simulink model "VirtualVehicle_lab2"  (R2021a)
settings: Solver=VariableStepAuto  StartTime=0.0  StopTime=30  MaxStep=0.002  RelTol=1e-3
libraries: PlantLibrary x1
settings Model: Creator=Rocksmithed  LastModifiedBy=Rocksmithed
settings ExplorerConfigSet: InternalSimMechanicsExplorerSettings="<ExplorerConfiguration><canonicalview>default</canonicalview><AnimationSetting><BasePlaybackSpeed>1.0</BasePlaybackSpeed><PlaybackSpeedFactor>1.0</PlaybackSpeedFactor></AnimationSetting><TilePanel><TileInfo><Tiles Columns=\"1\" Count=\"2\" Rows=\"2\"><Column Weight=\"1\"/><Row Weight=\"0.4997\"/><Row Weight=\"0.5003\"/><Tile Height=\"1\" Width=\"1\" X=\"0\" Y=\"0\"/><Tile Height=\"1\" Width=\"1\" X=\"0\" Y=\"1\"/></Tiles></TileInfo><SceneInfo><SceneViewer><BGColor><R>0.800000011920928955</R><G>0.800000011920928955</G><B>0.800000011920928955</B></BGColor><Camera><DoPerspective>on</DoPerspective><Position><X>442.389269826050509</X><Y>-6</Y><Z>6.75</Z></Position><Center><X>441.815693389699447</X><Y>-5.37249312840286741</Y><Z>6.22345921548163616</Z></Center><Up><X>0</X><Y>0</Y><Z>1</Z></Up><ViewLimDist>1</ViewLimDist><YLim>0.466307658154998583</YLim><XLim>1.37909215060664225</XLim></Camera></SceneViewer><SceneViewer><BGColor><R>0.800000011920928955</R><G>0.800000011920928955</G><B>0.800000011920928955</B></BGColor><Camera><DoPerspective>on</DoPerspective><Position><X>435.489269826050531</X><Y>-15</Y><Z>8.3066149444976863e-16</Z></Position><Center><X>435.489269826050531</X><Y>-14</Y><Z>6.08616889524737322e-16</Z></Center><Up><X>0</X><Y>0</Y><Z>1</Z></Up><ViewLimDist>1</ViewLimDist><YLim>0.466307658154998583</YLim><XLim>1.37741849508406133</XLim></Camera></SceneViewer></SceneInfo></TilePanel><MechEditorPanel><Cameras><Camera><Id>Camera1</Id><Value><Name>Camera1</Name><NativeCamera><PositionTrackingFeature>Vehicle_and_road.camera.R</PositionTrackingFeature><CenterTrackingFeature>Vehicle_and_road.camera.R</CenterTrackingFeature><UpVectorTrackingFeature>Vehicle_and_road.World_Frame.W</UpVectorTrackingFeature><CenterTrackingOrigin>off</CenterTrackingOrigin><CenterTrackingDirection>-Z</CenterTrackingDirection><UpVectorTrackingDirection>+Z</UpVectorTrackingDirection></NativeCamera></Value></Camera><Camera><Id>Camera2</Id><Value><Name>Camera2</Name><NativeCamera><PositionTrackingFeature>Vehicle_and_road.camera1.R</PositionTrackingFeature><CenterTrackingFeature>Vehicle_and_road.camera1.R</CenterTrackingFeature><UpVectorTrackingFeature>Vehicle_and_road.World_Frame.W</UpVectorTrackingFeature><CenterTrackingOrigin>off</CenterTrackingOrigin><CenterTrackingDirection>-Z</CenterTrackingDirection><UpVectorTrackingDirection>+Z</UpVectorTrackingDirection></NativeCamera></Value></Camera></Cameras><GfxPanelCameraMap><MapElement CameraMLId=\"Camera1\" GfxPanelIndex=\"0\"/><MapElement CameraMLId=\"Camera2\" GfxPanelIndex=\"1\"/></GfxPanelCameraMap><VideoCreator><PlaybackSpeedRatio>1.0</PlaybackSpeedRatio><FrameRate>30</FrameRate><VideoFormat>Motion JPEG AVI</VideoFormat><FrameSize>auto</FrameSize></VideoCreator></MechEditorPanel></ExplorerConfiguration>"

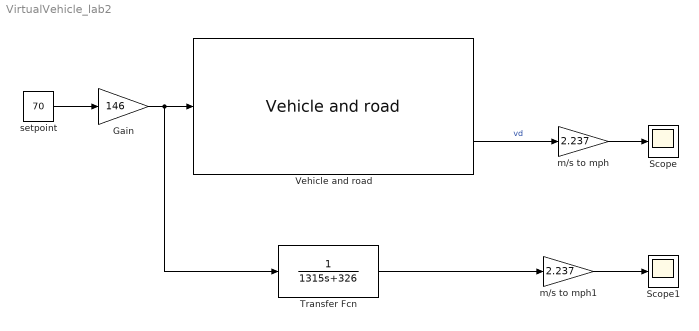
== system VirtualVehicle_lab2 ==
  Gain : Gain  Gain=146
  Scope : Scope
  Scope1 : Scope
  Transfer Fcn : TransferFcn  Denominator=[1315 326]
  Vehicle and road : PlantLibrary/Vehicle and road  MaxF=14800.0  brkok=on  dtype=none  randbumps=on  h=50  bumpspace=68.0
  m/s to mph : Gain  Gain=2.237
  m/s to mph1 : Gain  Gain=2.237
  setpoint : Constant  Value=70
  wires:
  setpoint/1 -> Gain/1
  Gain/1 -> Transfer Fcn/1, Vehicle and road/1
  Vehicle and road/2 -> m/s to mph/1  "vd"
  m/s to mph/1 -> Scope/1
  Transfer Fcn/1 -> m/s to mph1/1
  m/s to mph1/1 -> Scope1/1
